simulink model "ex02_multiregion_sim"  (R2017a)
settings: Solver=ode23s  StartTime=0.0  StopTime=8  RelTol=1e-3
values from neighbouring files (symbols this model uses):
  A = [0 1;0 0]    [ex01_linear_state_and_input_constraints.m]    (also in ex02_multiregion.m = kron(eye(2),[0 1;0 0]); ex02_polyhedral.m = kron(eye(2),[0 1;0 0]))
  B = [0;1]    [ex01_linear_state_and_input_constraints.m]    (also in ex02_multiregion.m = kron(eye(2),[0;1]); ex02_polyhedral.m = kron(eye(2),[0;1]))
  F = [-w^2 -2*z*w]    [ex01_linear_state_and_input_constraints.m]    (also in ex02_multiregion.m = kron(eye(2),[-w^2 -2*xi*w]); ex02_polyhedral.m = kron(eye(2),[-w^2 -2*xi*w]))
  G = w^2    (= 100)    [ex01_linear_state_and_input_constraints.m]    (also in ex02_multiregion.m = kron(eye(2),w^2); ex02_polyhedral.m = kron(eye(2),w^2))
  x0 = [0 0]'    [ex01_linear_state_and_input_constraints.m]    (also in ex02_multiregion.m = [-.7 0 -.7 0]'; ex02_polyhedral.m = [-.7 0 -.7 0]')
undefined symbols (not defined in the file): kappa, sys
libraries: ERG_lib x1
settings Model: Creator=Admin  LastModifiedBy=Admin

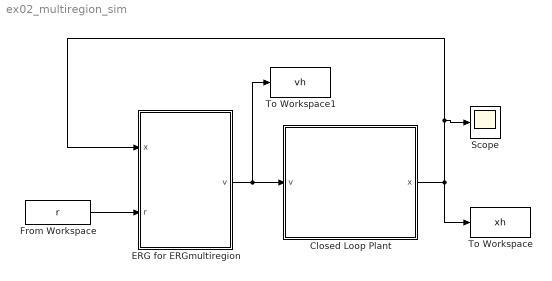
== system ex02_multiregion_sim ==
  Closed Loop Plant : Subsystem
  ERG for ERGmultiregion : Subsystem  mask(ERG with ERGmultiregion){sys_param=sys, eta_param=0.001, kappa_param=kappa}
      mask prompts: sys_param "ERGsys object:"; eta_param "eta:"; kappa_param "Gain (kappa):"
      mask help: This block is an Explicit Reference Governor for the case of union of convex polyhedral regions.
      mask Display:
      | port_label('input',1,'x')
      | port_label('input',2,'r')
      | port_label('output',1,'v')
  From Workspace : FromWorkspace  VariableName=r
  Scope : Scope
  To Workspace : ToWorkspace  VariableName=xh  SaveFormat=Timeseries  SampleTime=-1
  To Workspace1 : ToWorkspace  VariableName=vh  SaveFormat=Timeseries  SampleTime=-1
  wires:
  Closed Loop Plant/1(x) -> To Workspace/1, ERG for ERGmultiregion/1(x), Scope/1
  From Workspace/1 -> ERG for ERGmultiregion/2(r)
  ERG for ERGmultiregion/1(v) -> Closed Loop Plant/1(v), To Workspace1/1

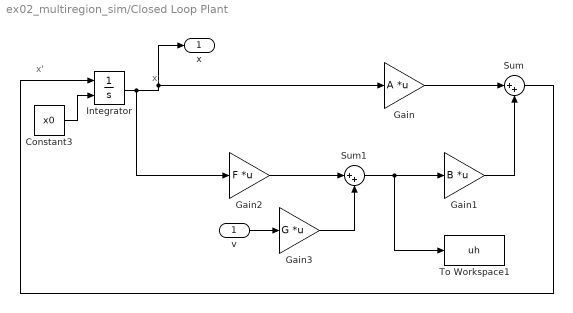
== system ex02_multiregion_sim/Closed Loop Plant ==
  note: x'
  note: x
  v : Inport
  Constant3 : Constant  Value=x0  VectorParams1D=off
  Gain : Gain  Gain=A  Multiplication=Matrix(K*u)
  Gain1 : Gain  Gain=B  Multiplication=Matrix(K*u)
  Gain2 : Gain  Gain=F  Multiplication=Matrix(K*u)
  Gain3 : Gain  Gain=G  Multiplication=Matrix(K*u)
  Integrator : Integrator  InitialConditionSource=external  InitialCondition=x0
  Sum : Sum  Inputs=|++
  Sum1 : Sum  Inputs=|++
  To Workspace1 : ToWorkspace  VariableName=uh  SaveFormat=Timeseries  SampleTime=-1
      settings: Save2DSignal=2-D array (concatenate along first dimension)
  x : Outport
  wires:
  Gain2/1 -> Sum1/1
  Gain3/1 -> Sum1/2
  Sum1/1 -> Gain1/1, To Workspace1/1
  Integrator/1 -> Gain2/1, x/1, Gain/1
  Sum/1 -> Integrator/1
  Gain1/1 -> Sum/2
  Constant3/1 -> Integrator/2
  Gain/1 -> Sum/1
  v/1 -> Gain3/1

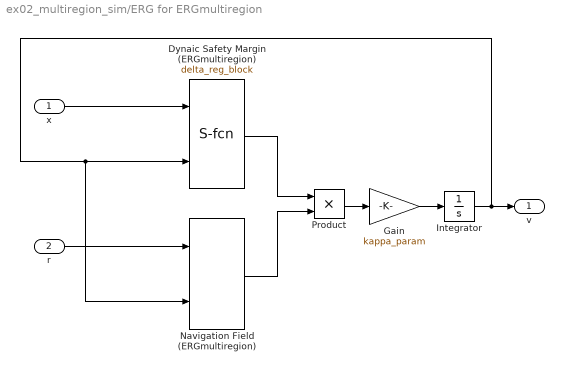
== system ex02_multiregion_sim/ERG for ERGmultiregion ==
  x : Inport
  r : Inport  Port=2
  Dynaic Safety Margin (ERGmultiregion) : M-S-Function  FunctionName=delta_reg_block  Parameters=system_param  mask(Dynamic Safety Margin for ERGmultiregion){system_param=sys_param}
      mask prompts: system_param "ERGsystem object:"
      mask help: This block calculates the Dynamic Safety Margin for an ERGsystem with an ERGmultiregion.
      mask Display:
      | port_label('input',1,'x')
      | port_label('input',2,'v')
      | port_label('output',1,'delta')
  Gain : Gain  Gain=kappa_param
  Integrator : Integrator  InitialCondition=sys_param.C*x0
  Navigation Field (ERGmultiregion) : ERG_lib/Navigation Field (ERGmultiregion)  system_param=sys_param  eta_param=eta_param
  Product : Product
  v : Outport
  wires:
  Product/1 -> Gain/1
  Gain/1 -> Integrator/1
  Dynaic Safety Margin (ERGmultiregion)/1 -> Product/1
  Navigation Field (ERGmultiregion)/1 -> Product/2
  x/1 -> Dynaic Safety Margin (ERGmultiregion)/1
  Integrator/1 -> Navigation Field (ERGmultiregion)/2, Dynaic Safety Margin (ERGmultiregion)/2, v/1
  r/1 -> Navigation Field (ERGmultiregion)/1
